simulink model "simulink5"  (R2017a)
settings: Solver=VariableStepAuto  StartTime=0.0  StopTime=2500  RelTol=1e-3
libraries: cstblocks x5
settings Model: Creator=Night_Fury  LastModifiedBy=Havoc

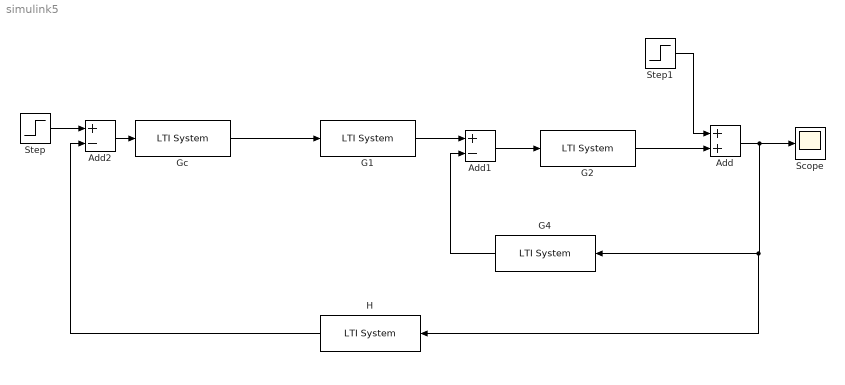
== system simulink5 ==
  Add : Sum
  Add1 : Sum  Inputs=+-
  Add2 : Sum  Inputs=+-
  G1 : cstblocks/LTI System  sys=tf([1],[1 1])  IC=[]
  G2 : cstblocks/LTI System  sys=tf([1],[1 1 8])  IC=[]
  G4 : cstblocks/LTI System  sys=tf([10],[2 1])  IC=[]
  Gc : cstblocks/LTI System  sys=tf([20],[1 1])  IC=[]
  H : cstblocks/LTI System  sys=tf(5,[1 0])  IC=[]
  Scope : Scope
  Step : Step  Time=0  SampleTime=0
  Step1 : Step  Time=0  SampleTime=0
  wires:
  Gc/1 -> G1/1
  G1/1 -> Add1/1
  Add1/1 -> G2/1
  G2/1 -> Add/2
  Step1/1 -> Add/1
  Add/1 -> H/1, G4/1, Scope/1
  G4/1 -> Add1/2
  Add2/1 -> Gc/1
  H/1 -> Add2/2
  Step/1 -> Add2/1
